simulink model "CTRL_LO_ST3_test"  (R2023b)
settings: Solver=VariableStepAuto  StartTime=0.0  StopTime=10.0  RelTol=1e-3
libraries: CTRL_LO_ST3 x1
settings Model: Creator=blatak  LastModifiedBy=blatak

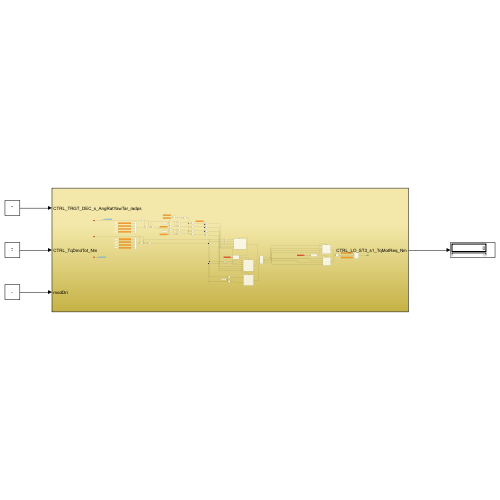
[thumbnail: Simulink's stored preview of the top-level diagram]
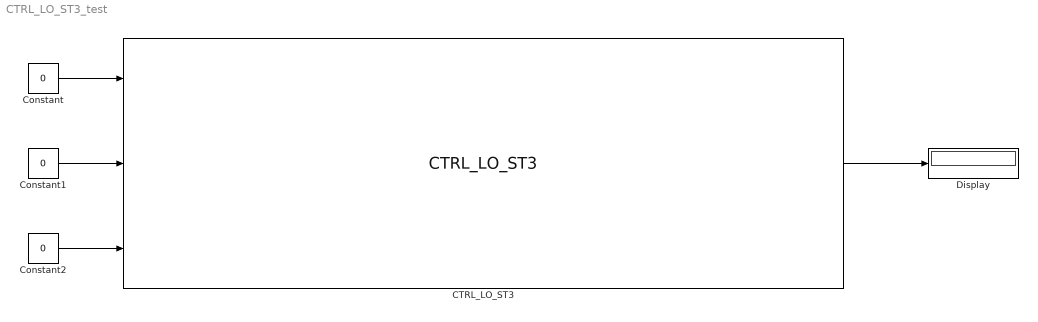
== system CTRL_LO_ST3_test ==
  CTRL_LO_ST3 : CTRL_LO_ST3/CTRL_LO_ST3  SystemSampleTime=-1  VariantActivationTime=update diagram  AllowFlexibleInterface=on  Latency=0  AutoFrameSizeCalculation=off
  Constant : Constant  Value=0  OutDataTypeStr=single
  Constant1 : Constant  Value=0  OutDataTypeStr=single
  Constant2 : Constant  Value=0  OutDataTypeStr=single
  Display : Display
  wires:
  Constant/1 -> CTRL_LO_ST3/1
  Constant1/1 -> CTRL_LO_ST3/2
  Constant2/1 -> CTRL_LO_ST3/3
  CTRL_LO_ST3/1 -> Display/1
